simulink model "slxMDCPFcnDemo"  (R2016a)
settings: Solver=ode5  StartTime=0.0  StopTime=inf  FixedStep=.001  RelTol=1e-3
settings Model: SimulationMode=external  Creator=julianleland  LastModifiedBy=julianleland
settings HardwareCC: ProdBitPerLong=64  ProdLargestAtomicFloat=None  ProdHWDeviceType=Intel->x86-64  TargetBitPerLong=64  TargetBitPerPointer=64  TargetIntDivRoundTo=Zero  TargetEndianess=LittleEndian  TargetWordSize=64  TargetHWDeviceType=Intel->x86-64
settings RTWCC: SystemTargetFile=sldrt.tlc  TemplateMakefile=sldrt.tmf  Description=Simulink Desktop Real-Time  RTWCompilerOptimization=on
settings CodeAppCC: MaxIdLength=95
settings SimulinkDesktopRealTimeCC: TargetPreCompLibLocation=/Applications/MATLAB_R2016a.app/toolbox/sldrt/lib/maci64  TargetLangStandard=C89/C90 (ANSI)  SupportVariableSizeSignals=off
settings ConfigComp: DVTestSuiteOptimization=CombinedObjectives (Nonlinear Extended)

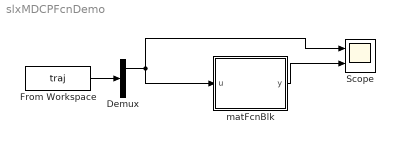
== system slxMDCPFcnDemo ==
  Demux : Demux  Outputs=2
  From Workspace : FromWorkspace  VariableName=traj  SampleTime=0
  Scope : Scope  NumInputPorts=2
  matFcnBlk : MATLAB Function  RequirementInfo="{}  %GIDa_c862cf31_d227_4f8c_b902_a0db74e02a20"  TreatAsAtomicUnit=on
  wires:
  matFcnBlk/1(y) -> Scope/2
  From Workspace/1 -> Demux/1
  Demux/1 -> matFcnBlk/1(u), Scope/1

== matlab function slxMDCPFcnDemo/matFcnBlk ==
  data: y output; robot parameter; u input
function y  = divide0p1(robot, u)
%#codegen

y = raw2joint_at40gw(robot,u);
%y = divide0p1_alt(u);
